simulink model "transcriptional_regulation"  (R2021b)
settings: Solver=VariableStepAuto  StartTime=0.0  StopTime=10  RelTol=1e-3
undefined symbols (not defined in the file): control, K_pp, ki, Kp, kr_pp
settings Model: Creator=UTENTE  LastModifiedBy=UTENTE

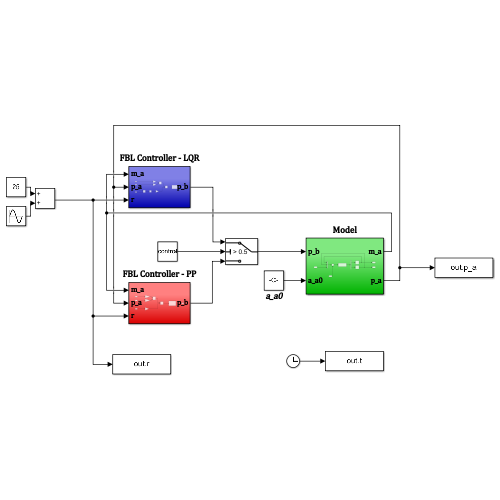
[thumbnail: Simulink's stored preview of the top-level diagram]
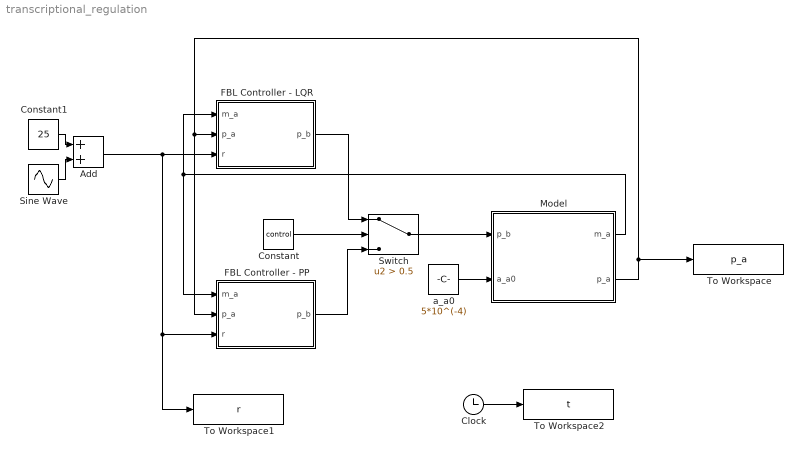
== system transcriptional_regulation ==
  Add : Sum
  Clock : Clock
  Constant : Constant  Value=control
  Constant1 : Constant  Value=25
  FBL Controller - LQR : Subsystem
  FBL Controller - PP : Subsystem
  Model : Subsystem
  Sine Wave : Sin  Frequency=0.01  SampleTime=0
  Switch : Switch  Criteria=u2 > Threshold  Threshold=0.5
  To Workspace : ToWorkspace  VariableName=p_a  SampleTime=-1
  To Workspace1 : ToWorkspace  VariableName=r  SampleTime=-1
  To Workspace2 : ToWorkspace  VariableName=t  SampleTime=-1
  a_a0 : Constant  Value=5*10^(-4)
  wires:
  Model/2(p_a) -> FBL Controller - PP/2(p_a), FBL Controller - LQR/2(p_a), To Workspace/1
  Add/1 -> To Workspace1/1, FBL Controller - PP/3(r), FBL Controller - LQR/3(r)
  a_a0/1 -> Model/2(a_a0)
  FBL Controller - PP/1(p_b) -> Switch/3
  Constant/1 -> Switch/2
  Clock/1 -> To Workspace2/1
  Switch/1 -> Model/1(p_b)
  Model/1(m_a) -> FBL Controller - LQR/1(m_a), FBL Controller - PP/1(m_a)
  Constant1/1 -> Add/1
  Sine Wave/1 -> Add/2
  FBL Controller - LQR/1(p_b) -> Switch/1

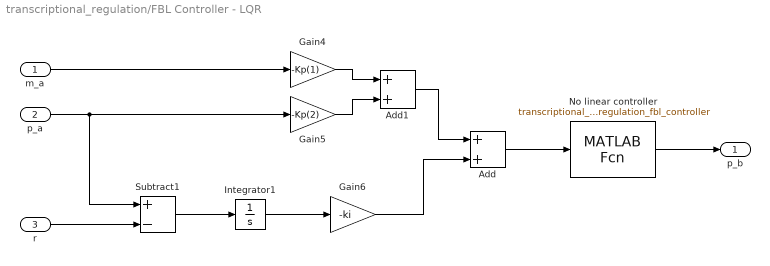
== system transcriptional_regulation/FBL Controller - LQR ==
  m_a : Inport
  p_a : Inport  Port=2
  r : Inport  Port=3
  Add : Sum
  Add1 : Sum
  Gain4 : Gain  Gain=-Kp(1)
  Gain5 : Gain  Gain=-Kp(2)
  Gain6 : Gain  Gain=-ki
  Integrator1 : Integrator  InitialCondition=-30
  No linear controller : MATLABFcn  MATLABFcn=transcriptional_regulation_fbl_controller  OutputDimensions=1
  Subtract1 : Sum  Inputs=+-
  p_b : Outport
  wires:
  Subtract1/1 -> Integrator1/1
  Gain5/1 -> Add1/2
  p_a/1 -> Subtract1/1, Gain5/1
  Gain4/1 -> Add1/1
  Add/1 -> No linear controller/1
  Gain6/1 -> Add/2
  r/1 -> Subtract1/2
  Add1/1 -> Add/1
  m_a/1 -> Gain4/1
  No linear controller/1 -> p_b/1
  Integrator1/1 -> Gain6/1

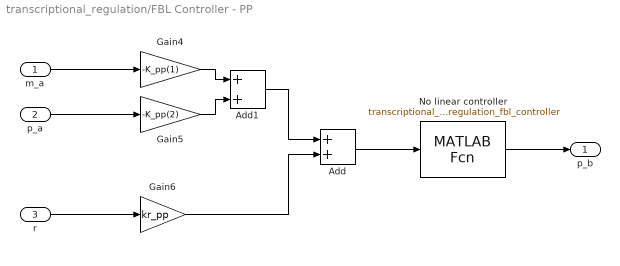
== system transcriptional_regulation/FBL Controller - PP ==
  m_a : Inport
  p_a : Inport  Port=2
  r : Inport  Port=3
  Add : Sum
  Add1 : Sum
  Gain4 : Gain  Gain=-K_pp(1)
  Gain5 : Gain  Gain=-K_pp(2)
  Gain6 : Gain  Gain=kr_pp
  No linear controller : MATLABFcn  MATLABFcn=transcriptional_regulation_fbl_controller  OutputDimensions=1
  p_b : Outport
  wires:
  Gain5/1 -> Add1/2
  p_a/1 -> Gain5/1
  Gain4/1 -> Add1/1
  Gain6/1 -> Add/2
  r/1 -> Gain6/1
  Add1/1 -> Add/1
  m_a/1 -> Gain4/1
  No linear controller/1 -> p_b/1
  Add/1 -> No linear controller/1

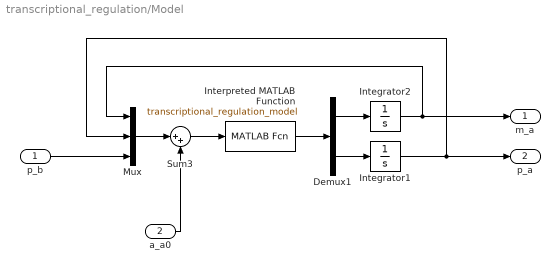
== system transcriptional_regulation/Model ==
  p_b : Inport
  a_a0 : Inport  Port=2
  Demux1 : Demux  Outputs=2
  Integrator1 : Integrator  InitialCondition=30
  Integrator2 : Integrator  InitialCondition=25
  Interpreted MATLAB Function : MATLABFcn  MATLABFcn=transcriptional_regulation_model  OutputDimensions=2
  Mux : Mux  Inputs=3
  Sum3 : Sum  Inputs=|++
  m_a : Outport
  p_a : Outport  Port=2
  wires:
  Sum3/1 -> Interpreted MATLAB Function/1
  Interpreted MATLAB Function/1 -> Demux1/1
  Mux/1 -> Sum3/1
  a_a0/1 -> Sum3/2
  Demux1/2 -> Integrator1/1
  p_b/1 -> Mux/3
  Integrator2/1 -> Mux/1, m_a/1
  Integrator1/1 -> Mux/2, p_a/1
  Demux1/1 -> Integrator2/1
